simulink model "sliding_rbf_adaptive"  (R2017b)
settings: Solver=VariableStepAuto  StartTime=0.0  StopTime=50  RelTol=1e-3
settings Model: Creator=SAZGARPARDAZ1  LastModifiedBy=SAZGARPARDAZ1

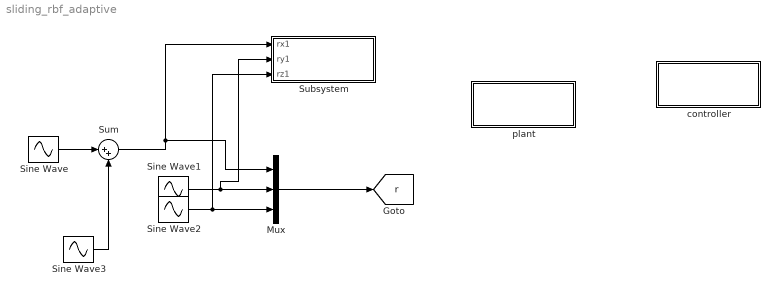
== system sliding_rbf_adaptive ==
  Mux : Mux  Inputs=3
  Sine Wave : Sin  Frequency=10  SampleTime=0
  Sine Wave1 : Sin  Amplitude=1.2  Frequency=30  SampleTime=0
  Sine Wave2 : Sin  Amplitude=1.5  Frequency=50  SampleTime=0
  Sine Wave3 : Sin  Amplitude=0  Frequency=15  SampleTime=0
  Subsystem : Subsystem
  Sum : Sum  Inputs=|++
  "controller " : Subsystem
  plant : Subsystem
  tag scope: r=global
  wires:
  Mux/1 -> [r]
  Sine Wave1/1 -> Subsystem/2(ry1), Mux/2
  Sine Wave2/1 -> Subsystem/3(rz1), Mux/3
  Sine Wave/1 -> Sum/1
  Sine Wave3/1 -> Sum/2
  Sum/1 -> Mux/1, Subsystem/1("rx1 ")

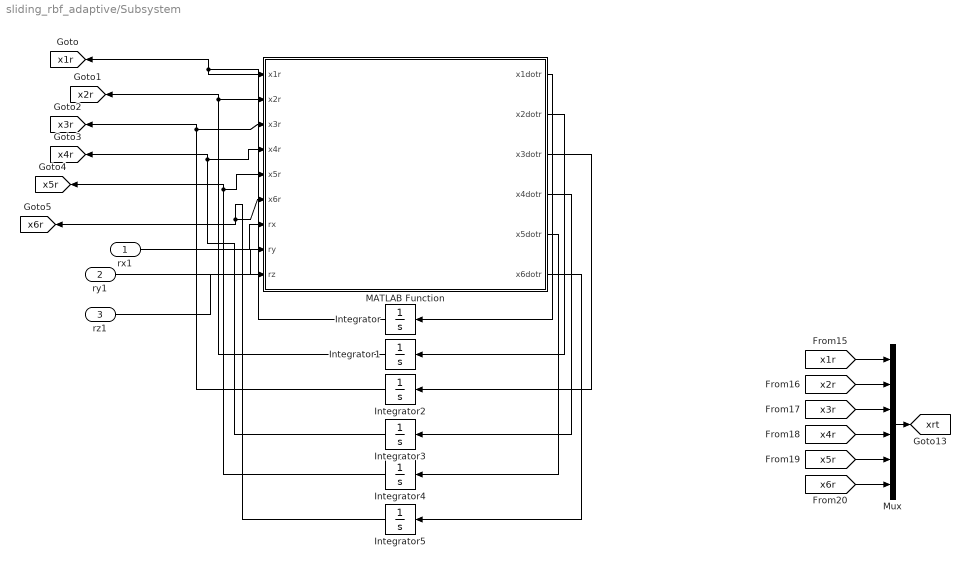
== system sliding_rbf_adaptive/Subsystem ==
  "rx1 " : Inport
  ry1 : Inport  Port=2
  rz1 : Inport  Port=3
  Integrator{,1..5} (6 alike) : Integrator
  MATLAB Function : MATLAB Function  TreatAsAtomicUnit=on
  Mux : Mux  Inputs=6
  tag scope: x1r=global, x2r=global, x3r=global, x4r=global, x5r=global, x6r=global, xrt=global
  wires:
  Integrator/1 -> [x1r], MATLAB Function/1(x1r)
  Integrator1/1 -> MATLAB Function/2(x2r), [x2r]
  Integrator2/1 -> [x3r], MATLAB Function/3(x3r)
  Integrator3/1 -> [x4r], MATLAB Function/4(x4r)
  Integrator4/1 -> [x5r], MATLAB Function/5(x5r)
  Integrator5/1 -> [x6r], MATLAB Function/6(x6r)
  "rx1 "/1 -> MATLAB Function/7(rx)
  ry1/1 -> MATLAB Function/8(ry)
  rz1/1 -> MATLAB Function/9(rz)
  MATLAB Function/1(x1dotr) -> Integrator/1
  MATLAB Function/2(x2dotr) -> Integrator1/1
  MATLAB Function/3(x3dotr) -> Integrator2/1
  MATLAB Function/4(x4dotr) -> Integrator3/1
  MATLAB Function/5(x5dotr) -> Integrator4/1
  MATLAB Function/6(x6dotr) -> Integrator5/1
  [x6r] -> Mux/6
  Mux/1 -> [xrt]
  [x5r] -> Mux/5
  [x4r] -> Mux/4
  [x1r] -> Mux/1
  [x3r] -> Mux/3
  [x2r] -> Mux/2

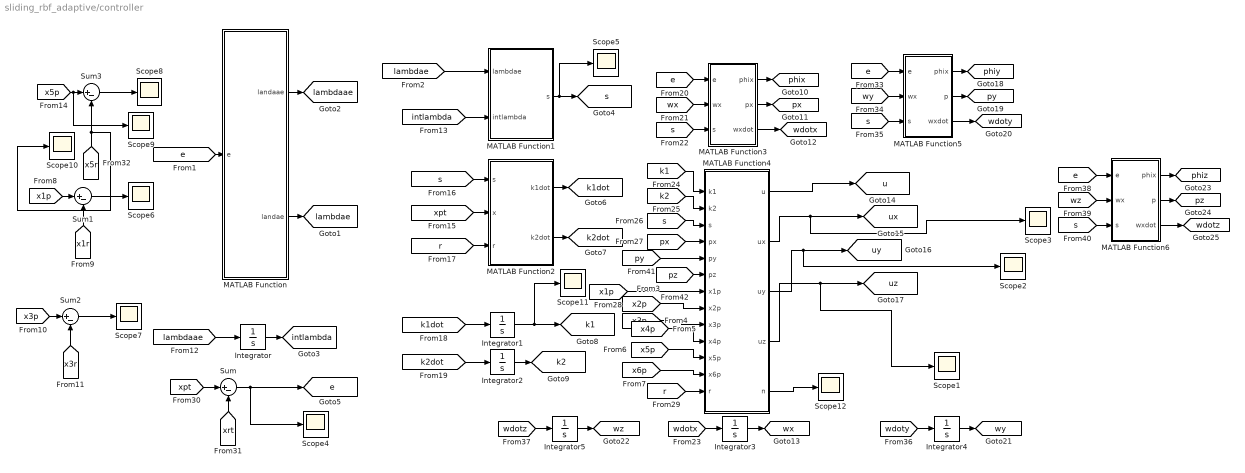
== system sliding_rbf_adaptive/controller  ==
  Integrator : Integrator  InitialCondition=[0;0;0;0;0;0]
  Integrator1 : Integrator  InitialCondition=[1380.15 87.719 105.2632;87.7193 1233 122.8070;105.2632 122.8070 1050.84;.0226 8.9978 3.6023;9.0036 .0362 5.3953;3.5964 5.4047 .0471]
  Integrator2 : Integrator  InitialCondition=eye(3)
  Integrator3 : Integrator  InitialCondition=[0.1;0.1;0.1]
  Integrator4 : Integrator  InitialCondition=[0.1;0.1;0.1]
  Integrator5 : Integrator  InitialCondition=[0.1;0.1;0.1]
  MATLAB Function : MATLAB Function  TreatAsAtomicUnit=on
  MATLAB Function1 : MATLAB Function  TreatAsAtomicUnit=on
  MATLAB Function2 : MATLAB Function  TreatAsAtomicUnit=on
  MATLAB Function3 : MATLAB Function  TreatAsAtomicUnit=on
  MATLAB Function4 : MATLAB Function  TreatAsAtomicUnit=on
  MATLAB Function5 : MATLAB Function  TreatAsAtomicUnit=on
  MATLAB Function6 : MATLAB Function  TreatAsAtomicUnit=on
  Scope{1..12} (12 alike) : Scope
  Sum{,1..3} (4 alike) : Sum  Inputs=|+-
  tag scope: e=global, intlambda=global, k1=global, k1dot=global, k2=global, k2dot=global, lambdaae=global, lambdae=global, phix=global, phiy=global, phiz=global, px=global, py=global, pz=global, s=global, u=global, ux=global, uy=global, uz=global, wdotx=global, wdoty=global, wdotz=global, wx=global, wy=global, wz=global
  wires:
  MATLAB Function/2(landae) -> [lambdae]
  MATLAB Function/1(landaae) -> [lambdaae]
  [lambdaae] -> Integrator/1
  Integrator/1 -> [intlambda]
  [intlambda] -> MATLAB Function1/2(intlambda)
  MATLAB Function1/1(s) -> Scope5/1, [s]
  [xpt] -> MATLAB Function2/2(x)
  [s] -> MATLAB Function2/1(s)
  [r] -> MATLAB Function2/3(r)
  MATLAB Function2/1(k1dot) -> [k1dot]
  MATLAB Function2/2(k2dot) -> [k2dot]
  Integrator1/1 -> Scope11/1, [k1]
  [k1dot] -> Integrator1/1
  [k2dot] -> Integrator2/1
  Integrator2/1 -> [k2]
  [e] -> MATLAB Function3/1(e)
  MATLAB Function3/1(phix) -> [phix]
  MATLAB Function3/2(px) -> [px]
  MATLAB Function3/3(wxdot) -> [wdotx]
  [wx] -> MATLAB Function3/2(wx)
  [s] -> MATLAB Function3/3(s)
  [wdotx] -> Integrator3/1
  Integrator3/1 -> [wx]
  [k1] -> MATLAB Function4/1(k1)
  [k2] -> MATLAB Function4/2(k2)
  [s] -> MATLAB Function4/3(s)
  [px] -> MATLAB Function4/4(px)
  [x1p] -> MATLAB Function4/7(x1p)
  [r] -> MATLAB Function4/13(r)
  MATLAB Function4/1(u) -> [u]
  MATLAB Function4/2(ux) -> Scope3/1, [ux]
  MATLAB Function4/3(uy) -> Scope2/1, [uy]
  MATLAB Function4/4(uz) -> Scope1/1, [uz]
  [xpt] -> Sum/1
  [xrt] -> Sum/2
  Sum/1 -> Scope4/1, [e]
  [e] -> MATLAB Function/1(e)
  [lambdae] -> MATLAB Function1/1(lambdae)
  [x2p] -> MATLAB Function4/8(x2p)
  [x3p] -> MATLAB Function4/9(x3p)
  [x4p] -> MATLAB Function4/10(x4p)
  [x5p] -> MATLAB Function4/11(x5p)
  [x6p] -> MATLAB Function4/12(x6p)
  [x1p] -> Sum1/1
  [x1r] -> Sum1/2
  Sum1/1 -> Scope6/1
  [x3p] -> Sum2/1
  Sum2/1 -> Scope7/1
  [x3r] -> Sum2/2
  [x5p] -> Scope9/1, Sum3/1
  Sum3/1 -> Scope8/1
  [x5r] -> Scope10/1, Sum3/2
  MATLAB Function5/3(wxdot) -> [wdoty]
  MATLAB Function5/2(p) -> [py]
  [s] -> MATLAB Function5/3(s)
  [wy] -> MATLAB Function5/2(wx)
  [e] -> MATLAB Function5/1(e)
  MATLAB Function5/1(phix) -> [phiy]
  [wdoty] -> Integrator4/1
  Integrator4/1 -> [wy]
  Integrator5/1 -> [wz]
  [wdotz] -> Integrator5/1
  MATLAB Function6/1(phix) -> [phiz]
  [wz] -> MATLAB Function6/2(wx)
  [e] -> MATLAB Function6/1(e)
  [s] -> MATLAB Function6/3(s)
  MATLAB Function6/2(p) -> [pz]
  MATLAB Function6/3(wxdot) -> [wdotz]
  [py] -> MATLAB Function4/5(py)
  [pz] -> MATLAB Function4/6(pz)
  MATLAB Function4/5(n) -> Scope12/1

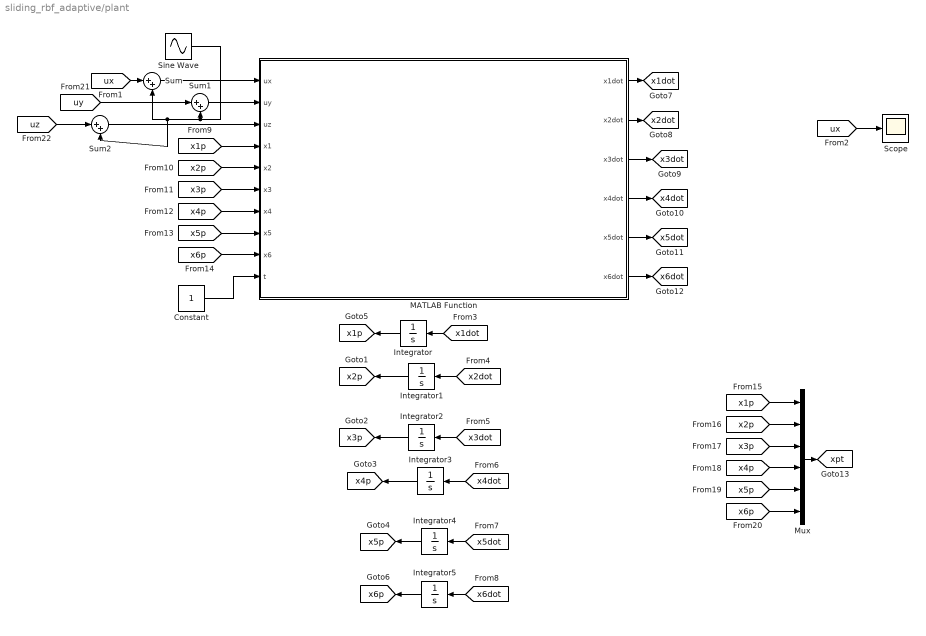
== system sliding_rbf_adaptive/plant ==
  Constant : Constant
  Integrator{,1..5} (6 alike) : Integrator
  MATLAB Function : MATLAB Function  TreatAsAtomicUnit=on
  Mux : Mux  Inputs=6
  Scope : Scope
  Sine Wave : Sin  SampleTime=0
  Sum : Sum  Inputs=|++
  Sum1 : Sum  Inputs=|++
  Sum2 : Sum  Inputs=|++
  tag scope: x1dot=global, x1p=global, x2dot=global, x2p=global, x3dot=global, x3p=global, x4dot=global, x4p=global, x5dot=global, x5p=global, x6dot=global, x6p=global, xpt=global
  wires:
  [ux] -> Scope/1
  [x1dot] -> Integrator/1
  Integrator/1 -> [x1p]
  [x2dot] -> Integrator1/1
  Integrator1/1 -> [x2p]
  [x3dot] -> Integrator2/1
  Integrator2/1 -> [x3p]
  [x4dot] -> Integrator3/1
  Integrator3/1 -> [x4p]
  [x5dot] -> Integrator4/1
  Integrator4/1 -> [x5p]
  [x6dot] -> Integrator5/1
  Integrator5/1 -> [x6p]
  MATLAB Function/1(x1dot) -> [x1dot]
  MATLAB Function/2(x2dot) -> [x2dot]
  MATLAB Function/3(x3dot) -> [x3dot]
  MATLAB Function/4(x4dot) -> [x4dot]
  MATLAB Function/5(x5dot) -> [x5dot]
  MATLAB Function/6(x6dot) -> [x6dot]
  [x1p] -> MATLAB Function/4(x1)
  [x2p] -> MATLAB Function/5(x2)
  [x3p] -> MATLAB Function/6(x3)
  [x4p] -> MATLAB Function/7(x4)
  [x5p] -> MATLAB Function/8(x5)
  [x6p] -> MATLAB Function/9(x6)
  Constant/1 -> MATLAB Function/10(t)
  [x1p] -> Mux/1
  [x2p] -> Mux/2
  [x3p] -> Mux/3
  [x4p] -> Mux/4
  [x5p] -> Mux/5
  [x6p] -> Mux/6
  Mux/1 -> [xpt]
  [ux] -> Sum/1
  Sum/1 -> MATLAB Function/1(ux)
  [uy] -> Sum1/1
  Sum1/1 -> MATLAB Function/2(uy)
  [uz] -> Sum2/1
  Sum2/1 -> MATLAB Function/3(uz)
  Sine Wave/1 -> Sum1/2, Sum2/2, Sum/2

== matlab function sliding_rbf_adaptive/Subsystem/MATLAB Function ==
  data: x1r input; x1dotr output; x2r input; x3r input; x4r input; x5r input; x6r input; x2dotr output; x3dotr output; x4dotr output; x5dotr output; x6dotr output; rx input; ry input; rz input
function [x1dotr, x2dotr, x3dotr, x4dotr, x5dotr, x6dotr] = fcn(x1r, x2r, x3r, x4r, x5r, x6r, rx, ry, rz)

x1dotr = x2r;
x2dotr = -45.0241*x1r + rx;
x3dotr = x4r;
x4dotr = -26.1121*x3r + ry;
x5dotr = x6r;
x6dotr = -17.3889*x5r + rz;

== matlab function sliding_rbf_adaptive/plant/MATLAB Function ==
  data: ux input; uy input; uz input; x1dot output; x1 input; x2 input; x3 input; x4 input; x5 input; x6 input; x2dot output; x3dot output; x4dot output; x5dot output; x6dot output; t input
function [x1dot, x2dot, x3dot, x4dot, x5dot, x6dot] = fcn(ux, uy, uz, x1, x2, x3, x4, x5, x6, t)


x1dot = x2;
x2dot = -1578.5241*x1 -.0251*x2 -97.4659*x3 - 9.9975*x4 - 116.9591*x5 -4.0025*x6 + ux;
x3dot = x4;
x4dot = -97.4659*x1 - 10.004*x2 - 1396.1121*x3 - 0.0402*x4 -136.4522*x5 -5.9948*x6 + uy;
x5dot = x6;
x6dot = -116.9591*x1 - 3.996*x2 - 136.4522*x3 - 6.0052*x4 + 1184.9889*x5 - .0523*x6 + uz;

== matlab function sliding_rbf_adaptive/controller /MATLAB Function ==
  data: landaae output; landae output; e input
function [landaae,landae] = fcn(e)

%intializing landa

Am = [0 1 0 0 0 0;-45.0241 0 0 0 0 0;0 0 0 1 0 0;0 0 -26.1121 0 0 0;0 0 0 0 0 1;0 0 0 0 -17.3889 0];
landa = diag([40,40,40,40,40,40]);
landaae = -landa*e;
landae = landa*e;

== matlab function sliding_rbf_adaptive/controller /MATLAB Function1 ==
  data: lambdae input; s output; intlambda input
function s = fcn(lambdae, intlambda)

s = lambdae - intlambda;

== matlab function sliding_rbf_adaptive/controller /MATLAB Function2 ==
  data: s input; k1dot output; x input; r input; k2dot output
function [k1dot, k2dot] = fcn(s, x, r)

%updating k1 and k2
%adaptive part
k1dot = zeros(6,3);
k2dot = zeros(3,3);

Q = .1*eye(3);
Bm = [0 0 0;1 0 0;0 0 0;0 1 0;0 0 0;0 0 1];
lambda = diag([40,40,40,40,40,40]);

k1dotp = - Q'*Bm'*(lambda)'*(s*x');
k1dot = k1dotp';
k2dot = - Q'*Bm'*(lambda)'*(s*r');

== matlab function sliding_rbf_adaptive/controller /MATLAB Function3 ==
  data: e input; phix output; wx input; s input; px output; wxdot output
function [phix, px, wxdot] = fcn(e , wx, s)

etha = 1;
q = [0;0;0];
qdot = [0;0;0];
q = [e(1)];
qdot = [e(2)];
mi = [-.1639 .7487 .5359;-0.3900 -.97 .9417];
sia = [.2;.2;.2];
phix = [0;0;0];
wxdot = [0;0;0];
k = 0;
px = 0;
d = [0;0];
for i = 1:3
    
    d = [q(1) - mi(1,i); qdot(1) - mi(2,i)];
    k = norm(d)
    phix(i) = exp(- k/(sia(i))^2);
end

px = (wx)'*phix;
wdotx = etha*norm(s)*phix;

== matlab function sliding_rbf_adaptive/controller /MATLAB Function4 ==
  data: k1 input; u output; k2 input; s input; px input; py input; pz input; x1p input; x2p input; x3p input; x4p input; x5p input; x6p input; r input; ux output; uy output; uz output; n output
function [u, ux, uy, uz, n] = fcn(k1, k2, s, px, py, pz, x1p,x2p,x3p,x4p,x5p,x6p, r)

ux = 0;
uy = 0;
uz = 0;
x = [x1p;x2p;x3p;x4p;x5p;x6p];
u = zeros(3,1);
s2 = [0;0;0];
s2 = [s(1);s(3);s(5)];
x1 = zeros(6,1);
u = (k1)'*x + k2*r ;
ux = u(1) - px*s2(1)/(norm(s2(1)) + 1);
uy = u(2) - py*s2(2)/(norm(s2(2)) + 1);
uz = u(3) - pz*s2(3)/(norm(s2(3)) + 1);
n = norm(s2)

== matlab function sliding_rbf_adaptive/controller /MATLAB Function5 ==
  data: e input; phix output; wx input; s input; p output; wxdot output
function [phix, p, wxdot] = fcn(e , wx, s)

etha = 5;
q = [0;0;0];
qdot = [0;0;0];
q = [e(3)];
qdot = [e(4)];
mi = [-.1639 .7487 .5359;-0.3900 -.97 .9417];
sia = [.2;.2;.2];
phix = [0;0;0];
wxdot = [0;0;0];
k = 0;
p = 0;
d = [0;0];
for i = 1:3
    
    d = [q(1) - mi(1,i); qdot(1) - mi(2,i)];
    k = norm(d)
    phix(i) = exp(- k/(sia(i))^2);
end

p = (wx)'*phix;
wxdot = etha*norm(s)*phix;

== matlab function sliding_rbf_adaptive/controller /MATLAB Function6 ==
  data: e input; phix output; wx input; s input; p output; wxdot output
function [phix, p, wxdot] = fcn(e , wx, s)

etha = 5;
q = [0;0;0];
qdot = [0;0;0];
q = [e(5)];
qdot = [e(6)];
mi = [-.1639 .7487 .5359;-0.3900 -.97 .9417];
sia = [.2;.2;.2];
phix = [0;0;0];
wxdot = [0;0;0];
k = 0;
p = 0;
d = [0;0];
for i = 1:3
    
    d = [q(1) - mi(1,i); qdot(1) - mi(2,i)];
    k = norm(d)
    phix(i) = exp(- k/(sia(i))^2);
end

p = (wx)'*phix;
wxdot = etha*norm(s)*phix;
